simulink model "CrashAlgo_TestEnvironment_Motorrad_v2"  (R2020b)
settings: Solver=FixedStepDiscrete  StartTime=0.0  StopTime=seconds(data.t(end))  FixedStep=0.01  MaxStep=0.2  RelTol=1e-3
values from neighbouring files (symbols this model uses):
  data = logFile.getSimulationData    [convertFiles2mat.m]    (also in startupThorsten.m)
undefined symbols (not defined in the file or in its folder): magnitude, Radix
libraries: dspstat3 x3, dspxfrm3 x2
settings Model: Creator=HNA3SI  LastModifiedBy=DAO1WA2
settings DebuggingCC: ReadBeforeWriteMsg=DisableAll  WriteAfterWriteMsg=DisableAll  WriteAfterReadMsg=DisableAll  ParameterPrecisionLossMsg=none
settings ModelReferenceCC: UpdateModelReferenceTargets=IfOutOfDate

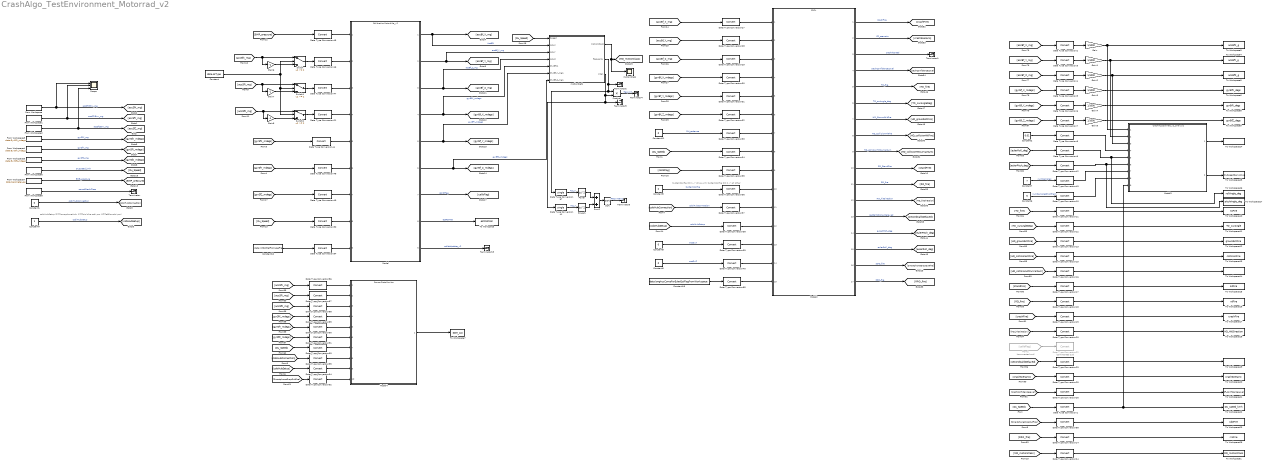
== system CrashAlgo_TestEnvironment_Motorrad_v2 ==
  note: cobiHubSetup (2==smarphoneHub, 1==bio bike cobi pro, 0==eBike cobi pro)
  note: SystemConfig == 1 -> drive unit, SystemConfig == 2 -> all other
  Constant : Constant  Value=data.osType
  Constant{1,3,8,11} (4 alike) : Constant  Value=0
  Constant10 : Constant  Value=data.InitRotMatFromLogFile
  Constant18 : Constant  Value=data.longAccCompForEulerEstFlagFromWorkspace
  Constant2 : Constant  Value=0.01
  Constant4 : Constant
  Constant5 : Constant  Value=2
  Constant6 : Constant  Value=5
  Constant7 : Constant  Value=7
  Data Type Conversion{1..20,23..26,42..43,58} (27 alike) : DataTypeConversion
  Data Type Conversion{21,27..40,44..50,54,85..95} (34 alike) : DataTypeConversion  RndMeth=Zero
  Data Type Conversion22 : DataTypeConversion  Commented=on
  Data Type Conversion41 : DataTypeConversion  OutDataTypeStr=single  RndMeth=Zero
  Data Type Conversion97 : DataTypeConversion  OutDataTypeStr=single  RndMeth=Zero
  From Workspace : FromWorkspace  VariableName=data.AccSfX_mg  SampleTime=0.01  Interpolate=off  ZeroCross=off  OutputAfterFinalValue=Setting to zero
  From Workspace1 : FromWorkspace  VariableName=data.AccSfY_mg  SampleTime=0.01  Interpolate=off  ZeroCross=off  OutputAfterFinalValue=Setting to zero
  From Workspace2 : FromWorkspace  VariableName=data.AccSfZ_mg  SampleTime=0.01  Interpolate=off  ZeroCross=off  OutputAfterFinalValue=Setting to zero
  From Workspace3 : FromWorkspace  VariableName=data.GyrSfX_mdegs  SampleTime=0.01  Interpolate=off  ZeroCross=off  OutputAfterFinalValue=Setting to zero
  From Workspace4 : FromWorkspace  VariableName=data.GyrSfY_mdegs  SampleTime=0.01  Interpolate=off  ZeroCross=off  OutputAfterFinalValue=Setting to zero
  From Workspace5 : FromWorkspace  VariableName=data.GyrSfZ_mdegs  SampleTime=0.01  Interpolate=off  ZeroCross=off  OutputAfterFinalValue=Setting to zero
  From Workspace6 : FromWorkspace  VariableName=data.speed_kmh  SampleTime=0.01  Interpolate=off  ZeroCross=off  OutputAfterFinalValue=Setting to zero
  From Workspace7 : FromWorkspace  VariableName=data.barometer_pa  SampleTime=0.01  Interpolate=off  ZeroCross=off  OutputAfterFinalValue=Setting to zero
  From Workspace8 : FromWorkspace  VariableName=data.crashClass  SampleTime=0.01  Interpolate=off  ZeroCross=off  OutputAfterFinalValue=Setting to zero
  From2 : From  Commented=on  GotoTag=calibFlag
  Gain{,1..5} (6 alike) : Gain  Gain=1/1000
  Gain6 : Gain  Gain=-1
  Gain7 : Gain  Gain=-1
  Gain8 : Gain  Gain=-1
  Model : ModelReference  ModelNameDialog=CalibrationMotorbike_v2.slx  SimulationMode=Normal  ModelReferenceVersion=4.9
  Model2 : ModelReference  ModelNameDialog=CRCL.slx  SimulationMode=Normal  ModelReferenceVersion=4.22
  Model3 : ModelReference  ModelNameDialog=CrashAlgoSchnee_v2_analysis.slx  SimulationMode=Normal  ModelReferenceVersion=4.11
  Model4 : ModelReference  ModelNameDialog=SensorDataMonitor.slx  SimulationMode=Normal  ModelReferenceVersion=4.4
  Power : Math  Operator=magnitude^2  SaturateOnIntegerOverflow=on
  Power1 : Math  Operator=magnitude^2  SaturateOnIntegerOverflow=on
  Product : Product
  Scope : Scope  NumInputPorts=3
  Sqrt : Sqrt  SaturateOnIntegerOverflow=on
  Sum2 : Sum
  Switch : Switch  Threshold=2
  Switch1 : Switch  Threshold=2
  Switch2 : Switch  Threshold=2
  Terminator{,1..5,15} (7 alike) : Terminator
  To Workspace : ToWorkspace  VariableName=estRotMat  SampleTime=-1
  To Workspace1 : ToWorkspace  VariableName=MD_motionClass  SampleTime=-1
  To Workspace10 : ToWorkspace  VariableName=toFire  SampleTime=-1
  To Workspace11 : ToWorkspace  VariableName=TO_curAngle  SampleTime=-1
  To Workspace12 : ToWorkspace  VariableName=groundHitFire  SampleTime=-1
  To Workspace13 : ToWorkspace  VariableName=collisionFire  SampleTime=-1
  To Workspace14 : ToWorkspace  VariableName=HD_CollisionCurVarSum  SampleTime=-1
  To Workspace15 : ToWorkspace  VariableName=sdFire  SampleTime=-1
  To Workspace16 : ToWorkspace  VariableName=rdFire  SampleTime=-1
  To Workspace17 : ToWorkspace  VariableName=crashFire  SampleTime=-1
  To Workspace18 : ToWorkspace  VariableName=HD_HitDirection  SampleTime=-1
  To Workspace19 : ToWorkspace  VariableName=SecondCalibrationDelayed  SampleTime=-1
  To Workspace20 : ToWorkspace  VariableName=crashScenario  SampleTime=-1
  To Workspace21 : ToWorkspace  VariableName=CF_confidenceLevel  SampleTime=-1
  To Workspace22 : ToWorkspace  VariableName=DU_speed_kmh  SampleTime=-1
  To Workspace23 : ToWorkspace  VariableName=sdoFire  SampleTime=-1
  To Workspace24 : ToWorkspace  VariableName=accImpulseXYsquaredSum  SampleTime=-1
  To Workspace25 : ToWorkspace  VariableName=DuSpeedDerivative  SampleTime=-1
  To Workspace26 : ToWorkspace  VariableName=rollAngle_deg  SampleTime=-1
  To Workspace27 : ToWorkspace  VariableName=pitchAngle_deg  SampleTime=-1
  To Workspace28 : ToWorkspace  VariableName=rroFire  SampleTime=-1
  To Workspace3 : ToWorkspace  VariableName=accBfX_g  SampleTime=-1
  To Workspace4 : ToWorkspace  VariableName=accBfY_g  SampleTime=-1
  To Workspace5 : ToWorkspace  VariableName=accBfZ_g  SampleTime=-1
  To Workspace6 : ToWorkspace  VariableName=gyrBfX_degs  SampleTime=-1
  To Workspace7 : ToWorkspace  VariableName=SDM_out  SampleTime=-1
  To Workspace8 : ToWorkspace  VariableName=gyrBfY_degs  SampleTime=-1
  To Workspace9 : ToWorkspace  VariableName=gyrBfZ_degs  SampleTime=-1
  motionClass : Scope
  motionDet1 : Subsystem
  wires:
  From Workspace6/1 -> [Du_Speed]  "DuSpeed_kmh"
  From Workspace1/1 -> [accSfY_mg], Scope/2  "accSfYEnv_mg"
  From Workspace/1 -> Scope/1, [accSfX_mg]  "accSfXEnv_mg"
  From Workspace2/1 -> [accSfZ_mg], Scope/3  "accSfZEnv_mg"
  From Workspace3/1 -> [gyrSfX_mdegs]  "gyrSfX_mg"
  From Workspace4/1 -> [gyrSfY_mdegs]  "gyrSfY_mg"
  From Workspace5/1 -> [gyrSfZ_mdegs]  "gyrSfZ_mg"
  Data Type Conversion29/1 -> Model2/3
  Constant18/1 -> Data Type Conversion85/1
  Model2/6 -> [TO_curAngleDeg]  "TO_curAngle_deg"
  Constant8/1 -> Data Type Conversion39/1  "accDuX"
  [gyrBf_Y_mdegs] -> Data Type Conversion31/1
  Data Type Conversion86/1 -> Model4/1
  Constant1/1 -> [cobiHubConnection]  "cobiHubConnection"
  Gain7/1 -> Switch1/3
  Model2/11 -> [RD_fire]  "RD_fire"
  Model2/9 -> [HD_collisionHitCurVarSum]  "HD_collisionHitCurVarSum"
  Data Type Conversion54/1 -> Model/9
  Model2/16 -> [SmartphoneDropOutFire]  "SDO_fire"
  Data Type Conversion48/1 -> Model/6
  [gyrBf_Z_mdegs] -> Data Type Conversion32/1
  Model2/1 -> [crashFire]  "CrashFire"
  Switch1/1 -> Data Type Conversion47/1
  [accBf_Y_mg] -> Data Type Conversion28/1
  Gain6/1 -> Switch/3
  [accSfZ_mg] -> Gain8/1, Switch2/1
  Data Type Conversion40/1 -> Model2/14
  Data Type Conversion27/1 -> Model2/1
  Data Type Conversion49/1 -> Model/7
  Model2/12 -> [HD_hitDirection]  "HD_hitDirection"
  Model2/4 -> [crashConfidenceLevel]  "crashConfidenceLevel"
  Data Type Conversion47/1 -> Model/3
  Model/7 -> [calibFlag]  "calibFlag"
  [calibFlag] -> Data Type Conversion35/1
  Constant/1 -> Switch2/2, Switch1/2, Switch/2
  Gain8/1 -> Switch2/3
  Data Type Conversion33/1 -> Model2/7
  Model2/2 -> [crashScenario]  "CP_scenario"
  Constant10/1 -> Data Type Conversion54/1
  Model2/14 -> [eulerPitch_deg]  "eulerPitch_deg"
  Model2/13 -> [secondCalibDelayed]  "secCalibDone Delayed"
  [accSfY_mg] -> Gain7/1, Switch1/1
  Data Type Conversion37/1 -> Model2/11
  Model/8 -> To Workspace/1  "estRotMat"
  Data Type Conversion32/1 -> Model2/6
  Model2/3 -> Terminator1/1  "crashAborted"
  [gyrSfX_mdegs] -> Data Type Conversion44/1
  Model2/15 -> [eulerRoll_deg]  "eulerRoll_deg"
  [Du_Speed] -> Data Type Conversion50/1
  Switch2/1 -> Data Type Conversion21/1
  Data Type Conversion28/1 -> Model2/2
  [gyrBf_X_mdegs] -> Data Type Conversion30/1
  Model/6 -> motionDet1/7(GyrBf_Z_mg1), [gyrBf_Z_mdegs]  "gyrBfZ_mdegs"
  Data Type Conversion35/1 -> Model2/9
  [BMP_pressure] -> Data Type Conversion45/1
  Data Type Conversion21/1 -> Model/4
  Constant5/1 -> Data Type Conversion36/1  "SystemConfig"
  Data Type Conversion36/1 -> Model2/10
  Data Type Conversion38/1 -> Model2/12
  [Du_Speed] -> Data Type Conversion93/1
  Switch/1 -> Data Type Conversion46/1
  Model2/5 -> [TO_fire]  "TO_fire"
  Constant11/1 -> Data Type Conversion33/1  "DU_cadence"
  [gyrSfZ_mdegs] -> Data Type Conversion91/1
  Model2/8 -> [HD_collisionHitFire]  "HD_CollisionHitFire"
  [cobiHubConnection] -> Data Type Conversion95/1
  [cobiHubSetup] -> Data Type Conversion94/1
  Model2/10 -> [standFire]  "SD_StandFire"
  Data Type Conversion46/1 -> Model/2
  Data Type Conversion88/1 -> Model4/3
  [accBf_Z_mg] -> Data Type Conversion29/1
  Model/9 -> Terminator15/1  "rotMatUpdate_v2"
  Model2/17 -> [RRO_fire]  "RRO_fire"
  Data Type Conversion94/1 -> Model4/9
  Constant3/1 -> Data Type Conversion40/1  "accDuZ"
  Data Type Conversion85/1 -> Model2/15
  Data Type Conversion50/1 -> Model/8
  Data Type Conversion93/1 -> Model4/7
  Data Type Conversion95/1 -> Model4/8
  Model2/7 -> [HD_groundHitFire]  "HD_GroundHitFire"
  Data Type Conversion44/1 -> Model/5
  [SmartphoneDropOutFire] -> Data Type Conversion92/1
  [Du_Speed] -> Data Type Conversion34/1
  [accSfZ_mg] -> Data Type Conversion88/1
  Data Type Conversion92/1 -> Model4/10
  Data Type Conversion31/1 -> Model2/5
  [accSfX_mg] -> Data Type Conversion86/1
  [accSfY_mg] -> Data Type Conversion87/1
  Data Type Conversion89/1 -> Model4/4
  Data Type Conversion30/1 -> Model2/4
  [accBf_X_mg] -> Data Type Conversion27/1
  [gyrSfY_mdegs] -> Data Type Conversion90/1
  [gyrSfY_mdegs] -> Data Type Conversion48/1
  Data Type Conversion34/1 -> Model2/8
  Data Type Conversion87/1 -> Model4/2
  Constant4/1 -> [cobiHubSetup]  "cobiHubSetup"
  Data Type Conversion45/1 -> Model/1
  [gyrSfZ_mdegs] -> Data Type Conversion49/1
  [accSfX_mg] -> Gain6/1, Switch/1
  [gyrSfX_mdegs] -> Data Type Conversion89/1
  Model4/1 -> To Workspace7/1
  Data Type Conversion90/1 -> Model4/5
  Data Type Conversion91/1 -> Model4/6
  Data Type Conversion39/1 -> Model2/13
  Data Type Conversion13/1 -> To Workspace12/1
  [gyrBf_Z_mdegs] -> Data Type Conversion7/1
  From2/1 -> Data Type Conversion22/1
  [Du_Speed] -> Data Type Conversion1/1
  [eulerPitch_deg] -> Data Type Conversion42/1
  Data Type Conversion11/1 -> To Workspace10/1
  [accBf_Y_mg] -> Data Type Conversion3/1
  Data Type Conversion2/1 -> Gain/1
  [gyrBf_Y_mdegs] -> Data Type Conversion6/1
  Gain2/1 -> To Workspace5/1, Model3/3
  Gain3/1 -> To Workspace6/1
  [crashScenario] -> Data Type Conversion25/1
  [accBf_Z_mg] -> Data Type Conversion4/1
  Data Type Conversion6/1 -> Gain4/1
  [TO_curAngleDeg] -> Data Type Conversion12/1
  [HD_collisionHitCurVarSum] -> Data Type Conversion16/1
  [eulerRoll_deg] -> Data Type Conversion9/1
  Data Type Conversion12/1 -> To Workspace11/1
  Data Type Conversion7/1 -> Gain5/1
  [TO_fire] -> Data Type Conversion11/1
  [accBf_X_mg] -> Data Type Conversion2/1
  Data Type Conversion43/1 -> Model3/7
  [crashFire] -> Data Type Conversion19/1
  Constant7/1 -> Data Type Conversion43/1  "numSamples"
  Constant2/1 -> Data Type Conversion8/1
  [gyrBf_X_mdegs] -> Data Type Conversion5/1
  Data Type Conversion5/1 -> Gain3/1
  Data Type Conversion3/1 -> Gain1/1
  Model3/2 -> To Workspace25/1
  [RRO_fire] -> Data Type Conversion14/1
  Gain/1 -> To Workspace3/1, Model3/1
  Data Type Conversion10/1 -> Model3/8
  [crashConfidenceLevel] -> Data Type Conversion26/1
  Data Type Conversion18/1 -> To Workspace16/1
  [HD_collisionHitFire] -> Data Type Conversion15/1
  [secondCalibDelayed] -> Data Type Conversion23/1
  Data Type Conversion1/1 -> To Workspace22/1, Model3/9
  Data Type Conversion9/1 -> To Workspace26/1, Model3/5
  Data Type Conversion58/1 -> To Workspace23/1
  [HD_groundHitFire] -> Data Type Conversion13/1
  Model3/1 -> To Workspace24/1
  [SmartphoneDropOutFire] -> Data Type Conversion58/1
  [HD_hitDirection] -> Data Type Conversion20/1
  Data Type Conversion26/1 -> To Workspace21/1
  Data Type Conversion8/1 -> Model3/4
  Data Type Conversion25/1 -> To Workspace20/1
  [standFire] -> Data Type Conversion17/1
  Data Type Conversion23/1 -> To Workspace19/1
  Data Type Conversion15/1 -> To Workspace13/1
  Constant6/1 -> Data Type Conversion10/1  "numSamplesShortTerm"
  Data Type Conversion20/1 -> To Workspace18/1
  Data Type Conversion19/1 -> To Workspace17/1
  [RD_fire] -> Data Type Conversion18/1
  Gain1/1 -> To Workspace4/1, Model3/2
  Data Type Conversion4/1 -> Gain2/1
  Data Type Conversion14/1 -> To Workspace28/1
  Gain5/1 -> To Workspace9/1
  Gain4/1 -> To Workspace8/1
  Data Type Conversion42/1 -> To Workspace27/1, Model3/6
  Data Type Conversion16/1 -> To Workspace14/1
  Data Type Conversion17/1 -> To Workspace15/1
  From Workspace7/1 -> [BMP_pressure]  "BME_pressure"
  From Workspace8/1 -> Terminator/1  "savedCrashClass"
  [cobiHubConnection] -> Data Type Conversion37/1  "cobiHubConnection"
  [cobiHubSetup] -> Data Type Conversion38/1  "cobiHubSetup"
  [MD_motionClass] -> Data Type Conversion24/1
  Data Type Conversion24/1 -> To Workspace1/1
  motionDet1/2(frequency) -> Data Type Conversion97/1, Product/1, Terminator2/1
  [Du_Speed] -> motionDet1/1(Speed)
  Data Type Conversion97/1 -> Power/1  "Acc_X"
  Power1/1 -> Sum2/2
  Data Type Conversion41/1 -> Power1/1  "Acc_Y"
  Sum2/1 -> Sqrt/1
  Sqrt/1 -> Terminator5/1  "FreqxInten2"
  Power/1 -> Sum2/1
  Model/4 -> motionDet1/5(GyrBfX1), [gyrBf_X_mdegs]  "gyrBfX_mdegs"
  Model/1 -> motionDet1/2(Acc_X), [accBf_X_mg]  "AccBfX"
  Product/1 -> Terminator4/1  "freqxInt"
  motionDet1/1(motionClass) -> motionClass/1, [MD_motionClass]
  Model/3 -> motionDet1/4(Acc_Z), [accBf_Z_mg]  "accBf_Z_mg"
  Model/5 -> motionDet1/6(GyrBf_Y_mg1), [gyrBf_Y_mdegs]  "gyrBfY_mdegs"
  motionDet1/3(Inten) -> Data Type Conversion41/1, Terminator3/1, Product/2
  Model/2 -> motionDet1/3(Acc_Y), [accBf_Y_mg]  "accBf_Y_mg"

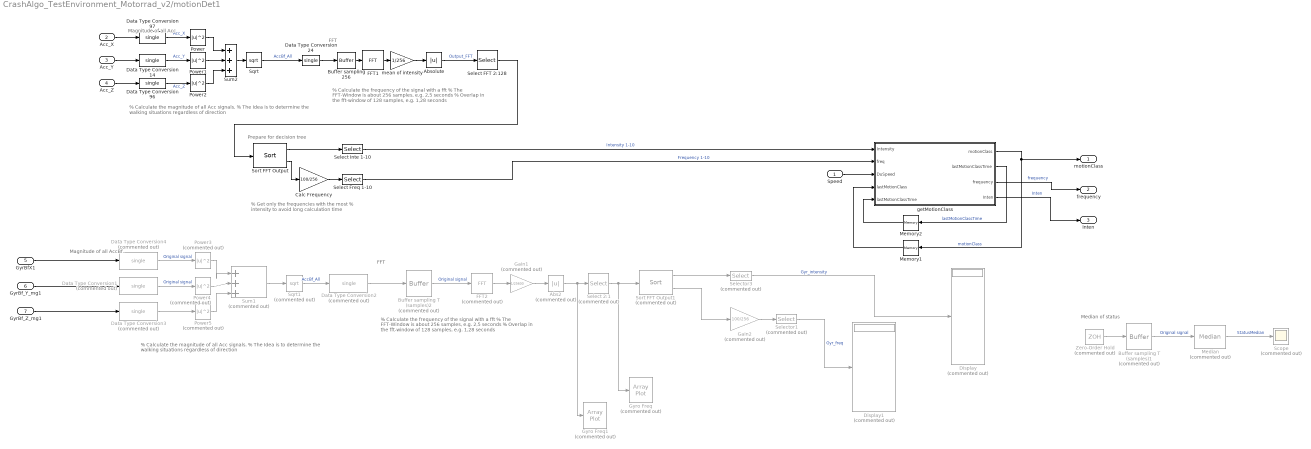
== system CrashAlgo_TestEnvironment_Motorrad_v2/motionDet1 ==
  note: Prepare for decision tree
  note: Magnitude of all AccBf.
  note: % Calculate the magnitude of all Acc signals.
      | % The Idea is to determine the walking situations regardless of direction
  note: FFT
  note: % Calculate the frequency of the signal with a fft
      | % The FFT-Window is about 256 samples, e.g. 2,5 seconds
      | % Overlap in the fft-window of 128 samples, e.g. 1,28 seconds
  note: Magnitude of all Acc
  note: % Calculate the magnitude of all Acc signals.
      | % The Idea is to determine the walking situations regardless of direction
  note: FFT
  note: % Calculate the frequency of the signal with a fft
      | % The FFT-Window is about 256 samples, e.g. 2,5 seconds
      | % Overlap in the fft-window of 128 samples, e.g. 1,28 seconds
  note: Median of status
  note: % Get only the frequencies with the most
      | % intensity to avoid long calculation time
  Speed : Inport
  Acc_X : Inport  Port=2
  Acc_Y : Inport  Port=3
  Acc_Z : Inport  Port=4
  GyrBfX1 : Inport  Port=5
  GyrBf_Y_mg1 : Inport  Port=6
  GyrBf_Z_mg1 : Inport  Port=7
  Abs2 : Abs  Commented=on
  Absolute : Abs
  "Buffer sampling 256 " : Buffer  N=256  V=128  OutputFrames=off
  Buffer sampling T (samples)1 : Buffer  Commented=on  N=39  V=19  OutputFrames=off
  Buffer sampling T (samples)2 : Buffer  Commented=on  N=256  V=128  OutputFrames=off
  Calc Frequency : Gain  Gain=100/256
  Data Type Conversion{1..4} (4 alike) : DataTypeConversion  Commented=on  OutDataTypeStr=single  RndMeth=Zero
  Data Type Conversion{14,24,96..97} (4 alike) : DataTypeConversion  OutDataTypeStr=single  RndMeth=Zero
  Display : Display  Commented=on
  Display1 : Display  Commented=on
  FFT1 : dspxfrm3/FFT  FFTImplementation=Radix-2  CompMethod=Table lookup  TableOpt=NEW  TableOptActive=Speed  BitRevOrder=off  Normalize=off  InheritFFTLength=on  FFTLength=256  WrapInput=off  roundingMode=Floor  overflowMode=off  firstCoeffDataTypeStr=Inherit: Same word length as input  firstCoeffLastDataTypeStr=Inherit: Same word length as input  outputMin=[]  outputMax=[]
  FFT2 : dspxfrm3/FFT  Commented=on  FFTImplementation=Radix-2  CompMethod=Table lookup  TableOpt=NEW  TableOptActive=Speed  BitRevOrder=off  Normalize=off  InheritFFTLength=on  FFTLength=256  WrapInput=off  roundingMode=Floor  overflowMode=off  firstCoeffDataTypeStr=Inherit: Same word length as input  firstCoeffLastDataTypeStr=Inherit: Same word length as input  outputMin=[]  outputMax=[]
  Gain1 : Gain  Commented=on  Gain=1/25600
  Gain2 : Gain  Commented=on  Gain=100/256
  Gyro Freq : ArrayPlot  Commented=on
  Gyro Freq1 : ArrayPlot  Commented=on
  Median : dspstat3/Median  Commented=on  sortAlg=Quick sort  directionMode=Entire input  dimension=1  roundingMode=Floor  overflowMode=off  accumDataTypeStr=Inherit: Same as product output  accumLastDataTypeStr=Inherit: Same as product output  outputDataTypeStr=Inherit: Same as accumulator  outputMin=[]  outputMax=[]  outputLastDataTypeStr=Inherit: Same as accumulator
      settings: SourceProductBaseCode=DS  allowOverrides=off
  Memory1 : Memory
  Memory2 : Memory
  Power : Math  Operator=magnitude^2  SaturateOnIntegerOverflow=on
  Power1 : Math  Operator=magnitude^2  SaturateOnIntegerOverflow=on
  Power2 : Math  Operator=magnitude^2  SaturateOnIntegerOverflow=on
  Power3 : Math  Commented=on  Operator=magnitude^2  SaturateOnIntegerOverflow=on
  Power4 : Math  Commented=on  Operator=magnitude^2  SaturateOnIntegerOverflow=on
  Power5 : Math  Commented=on  Operator=magnitude^2  SaturateOnIntegerOverflow=on
  Scope : Scope  Commented=on
  Select 2:1 : Selector  Commented=on  IndexOptions=Index vector (dialog)  Indices=2:128  OutputSizes=1
  Select FFT 2:128 : Selector  IndexOptions=Index vector (dialog)  Indices=2:128  OutputSizes=1
  Select Freq 1-10 : Selector  InputPortWidth=127  IndexOptions=Index vector (dialog)  Indices=1:10  OutputSizes=1
  Select Inte 1-10 : Selector  InputPortWidth=127  IndexOptions=Index vector (dialog)  Indices=1:10  OutputSizes=1
  Selector1 : Selector  Commented=on  InputPortWidth=127  IndexOptions=Index vector (dialog)  Indices=1:10  OutputSizes=1
  Selector3 : Selector  Commented=on  InputPortWidth=127  IndexOptions=Index vector (dialog)  Indices=1:10  OutputSizes=1
  Sort FFT Output : dspstat3/Sort  otype=Value and Index  dir=Descending  sortAlg=Quick sort  roundingMode=Floor  overflowMode=off  accumDataTypeStr=Inherit: Same as product output  accumLastDataTypeStr=Inherit: Same as product output
      settings: SourceProductBaseCode=DS
  Sort FFT Output1 : dspstat3/Sort  Commented=on  otype=Value and Index  dir=Descending  sortAlg=Quick sort  roundingMode=Floor  overflowMode=off  accumDataTypeStr=Inherit: Same as product output  accumLastDataTypeStr=Inherit: Same as product output
      settings: SourceProductBaseCode=DS
  Sqrt : Sqrt  SaturateOnIntegerOverflow=on
  Sqrt1 : Sqrt  Commented=on  SaturateOnIntegerOverflow=on
  Sum1 : Sum  Commented=on  Inputs=|+++
  Sum2 : Sum  Inputs=+++
  Zero-Order Hold : ZeroOrderHold  Commented=on  SampleTime=10e-2
  getMotionClass : MATLAB Function  TreatAsAtomicUnit=on
  mean of intensity : Gain  Gain=1/256
  motionClass : Outport
  frequency : Outport  Port=2
  Inten : Outport  Port=3
  wires:
  Selector1/1 -> Display1/1  "Gyr_freq"
  Gain1/1 -> Abs2/1
  FFT2/1 -> Gain1/1
  Buffer sampling T (samples)2/1 -> FFT2/1  "Original signal"
  Data Type Conversion2/1 -> Buffer sampling T (samples)2/1
  GyrBf_Z_mg1/1 -> Data Type Conversion3/1
  Power3/1 -> Sum1/1
  GyrBfX1/1 -> Data Type Conversion4/1
  GyrBf_Y_mg1/1 -> Data Type Conversion1/1
  Power4/1 -> Sum1/2
  Data Type Conversion1/1 -> Power4/1  "Original signal"
  Data Type Conversion4/1 -> Power3/1  "Original signal"
  Power5/1 -> Sum1/3
  Sum1/1 -> Sqrt1/1
  Data Type Conversion3/1 -> Power5/1
  Sqrt1/1 -> Data Type Conversion2/1  "AccBf_All"
  Abs2/1 -> Select 2:1/1, Gyro Freq1/1
  Sort FFT Output1/1 -> Selector3/1
  Sort FFT Output1/2 -> Gain2/1
  Selector3/1 -> Display/1  "Gyr_intensity"
  Select 2:1/1 -> Sort FFT Output1/1, Gyro Freq/1
  Gain2/1 -> Selector1/1
  Memory2/1 -> getMotionClass/5("lastMotionClassTime ")
  getMotionClass/2(lastMotionClassTime) -> Memory2/1  "lastMotionClassTime"
  Zero-Order Hold/1 -> Buffer sampling T (samples)1/1
  Median/1 -> Scope/1  "StatusMedian"
  Buffer sampling T (samples)1/1 -> Median/1  "Original signal"
  Select Freq 1-10/1 -> getMotionClass/2(freq)  "Frequency 1-10"
  Calc Frequency/1 -> Select Freq 1-10/1
  Select FFT 2:128/1 -> Sort FFT Output/1
  Select Inte 1-10/1 -> getMotionClass/1(Intensity)  "Intensity 1-10"
  Sort FFT Output/2 -> Calc Frequency/1
  Speed/1 -> getMotionClass/3(DuSpeed)
  Sort FFT Output/1 -> Select Inte 1-10/1
  getMotionClass/1(motionClass) -> motionClass/1, Memory1/1  "motionClass"
  Memory1/1 -> getMotionClass/4(lastMotionClass)
  Absolute/1 -> Select FFT 2:128/1  "Output_FFT"
  Sqrt/1 -> Data Type Conversion24/1  "AccBf_All"
  Data Type Conversion96/1 -> Power2/1  "Acc_Z"
  Sum2/1 -> Sqrt/1
  Power2/1 -> Sum2/3
  Data Type Conversion97/1 -> Power/1  "Acc_X"
  Data Type Conversion14/1 -> Power1/1  "Acc_Y"
  Power1/1 -> Sum2/2
  Acc_Y/1 -> Data Type Conversion14/1
  Acc_X/1 -> Data Type Conversion97/1
  Power/1 -> Sum2/1
  Acc_Z/1 -> Data Type Conversion96/1
  Data Type Conversion24/1 -> "Buffer sampling 256 "/1
  "Buffer sampling 256 "/1 -> FFT1/1
  FFT1/1 -> mean of intensity/1
  mean of intensity/1 -> Absolute/1
  getMotionClass/3(frequency) -> frequency/1  "frequency"
  getMotionClass/4(Inten) -> Inten/1  "Inten"

== matlab function CrashAlgo_TestEnvironment_Motorrad_v2/motionDet1/getMotionClass ==
  data: Intensity input; freq input; DuSpeed input; lastMotionClass input; motionClass output; lastMotionClassTime output; lastMotionClassTime input; frequency output; Inten output
function [motionClass, lastMotionClassTime, frequency, Inten] = getMotionClass(Intensity, freq, DuSpeed, lastMotionClass, lastMotionClassTime)
% status = -1;
for iFq = 1:5
    if Intensity(iFq) > 100
        lastMotionClassTime = 0;
        %         lastClassTime = 0;
        if freq(iFq) >= 7
            % high frequency (most likely driving), check with speed
            if DuSpeed < 5
                % high frequency but very low speed => sitting on motorbike and standing still
                motionClass = 0;
            else
                % there is movement
                motionClass = 2;
            end
            break
        elseif freq(iFq) >= 0.390625000 && freq(iFq) <= 2
            % walking, (most likely walking) check with speed
            if DuSpeed <=7 && DuSpeed > 0
                % walking speed
                motionClass = 1;
                break
            elseif DuSpeed == 0
                % no speed, propably standing
                motionClass = 0;
                break
            else
                % speed > 7 kmh => not walking => conflict => check next frequency
                motionClass = -1;
                continue;
            end
        elseif freq(iFq) > 2 && freq(iFq) <7
            % undeclared. Maybe walking and maybe driving. Double check with the spped. If the speed is bigger than 7 km/h than he must be driving.
            % If the speed's smaller than 7 km/h it should stay undeclared, he might be driving with no GPS-Signal (e.g. no speed) or walking
            if DuSpeed >= 7
                motionClass = 2;
                break;
            else
                motionClass = -1;
                continue;
            end
            
        elseif freq(iFq) < 0.3906 % undeclared f < 0.3906 Hz
            % not intended to get here
            % (sensor couldn't sense frequencies smaller than 0.396)
            motionClass = -2;
            break
        else
            % not intended to get here either; all usecases were defined in the
            % previous elseifs
            motionClass = lastMotionClass;
            break
        end
    else
        if DuSpeed >= 7
            motionClass = 2;
            break;
        elseif DuSpeed < 7 && DuSpeed > 0.1  
            motionClass = 1;
            break;
%             if lastMotionClassTime <=100
%                 lastMotionClassTime = lastMotionClassTime + 1;
%                 motionClass = lastMotionClass;
%             else
%                 lastMotionClassTime = 0;
%                 motionClass = 1;
%             end
%             continue
            break;
        else
            motionClass = 0;
        end
        lastMotionClassTime = 0;
    end
end
frequency = freq(iFq);
Inten = Intensity(iFq);
end

% statusAll = [statusAll status];
